simulink model "nid_cvst_what_nid_see"  (Simulink 10.0)
settings: Solver=FixedStepDiscrete  StartTime=0.0  StopTime=inf  RelTol=1e-3  EnableMultiTasking=on
libraries: nid_lib x5, viptextngfix x4, vipsnks x1
settings Model: Creator=tchikama  LastModifiedBy=bhisma
settings DataIOCC: LimitDataPoints=on  SignalLoggingSaveFormat=ModelDataLogs  SaveOutput=off
settings OptimizationCC: ExpressionDepthLimit=2147483647  SimCompilerOptimization=on
settings DebuggingCC: SolverPrmCheckMsg=warning  FcnCallInpInsideContextMsg=warning  StateNameClashWarn=warning
settings HardwareCC: ProdIntDivRoundTo=Zero  ProdEndianess=LittleEndian  ProdHWDeviceType=Generic->32-bit x86 compatible
settings RTWCC: RTWCompilerOptimization=on
settings CodeAppCC: MaxIdLength=95
settings GRTTargetCC: GeneratePreprocessorConditionals=Disable all
settings ConfigComp: CovExternalEMLEnable=off

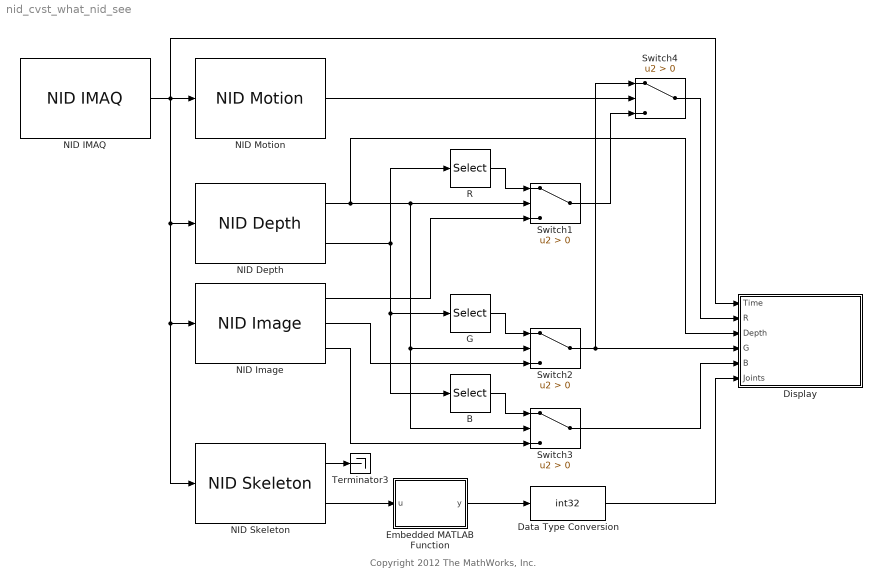
== system nid_cvst_what_nid_see ==
  note: Copyright 2012 The MathWorks, Inc.
  B : Selector  NumberOfDimensions=3  InputPortWidth=3  IndexOptions=Select all,Select all,Index vector (dialog)  Indices=1,2,3  OutputSizes=1,1,1
  Data Type Conversion : DataTypeConversion  OutDataTypeStr=int32
  Display : Subsystem  mask{text_color=[0 0 0]}
      mask prompts: text_color "Text Color (RGB)"
  Embedded MATLAB Function : MATLAB Function  TreatAsAtomicUnit=on
  G : Selector  NumberOfDimensions=3  InputPortWidth=3  IndexOptions=Select all,Select all,Index vector (dialog)  Indices=1,2,2  OutputSizes=1,1,1
  NID Depth : nid_lib/NID Depth  depthOutput=Depth  conv_XYZ_RW=off  viewer=on
  NID IMAQ : nid_lib/NID IMAQ  imaq_depth=on  imaq_motion=on  imaq_image=on  view_point=on  imaq_skeleton=on  imaq_ir=off  mirror_image=off  imaq_sample_time=1/30  res_fps=VGA (640x480): 30 FPS  needPsiPose=off  angle=0  angle_read=off  near_mode=off
  NID Image : nid_lib/NID Image  imageOutput=R/G/B
  NID Motion : nid_lib/NID Motion  viewer=off
  NID Skeleton : nid_lib/NID Skeleton  num_of_skeleton_tracking=1  conv_XYZ_RW=off  viewer=off
  R : Selector  NumberOfDimensions=3  InputPortWidth=3  IndexOptions=Select all,Select all,Index vector (dialog)  Indices=1,2,1  OutputSizes=1,1,1
  Switch{1..4} (4 alike) : Switch  Criteria=u2 > Threshold
  Terminator3 : Terminator
  wires:
  NID IMAQ/1 -> NID Motion/1, NID Depth/1, NID Skeleton/1, NID Image/1, Display/1(Time)
  R/1 -> Switch1/1
  NID Image/1 -> Switch1/3
  G/1 -> Switch2/1
  B/1 -> Switch3/1
  NID Image/2 -> Switch2/3
  NID Image/3 -> Switch3/3
  NID Depth/2 -> R/1, G/1, B/1
  NID Depth/1 -> Switch1/2, Switch2/2, Switch3/2, Display/3(Depth)
  Switch2/1 -> Switch4/1, Display/4(G)
  NID Motion/1 -> Switch4/2
  Switch1/1 -> Switch4/3
  Switch4/1 -> Display/2(R)
  Switch3/1 -> Display/5(B)
  NID Skeleton/1 -> Terminator3/1
  NID Skeleton/2 -> Embedded MATLAB Function/1(u)
  Embedded MATLAB Function/1(y) -> Data Type Conversion/1
  Data Type Conversion/1 -> Display/6(Joints)

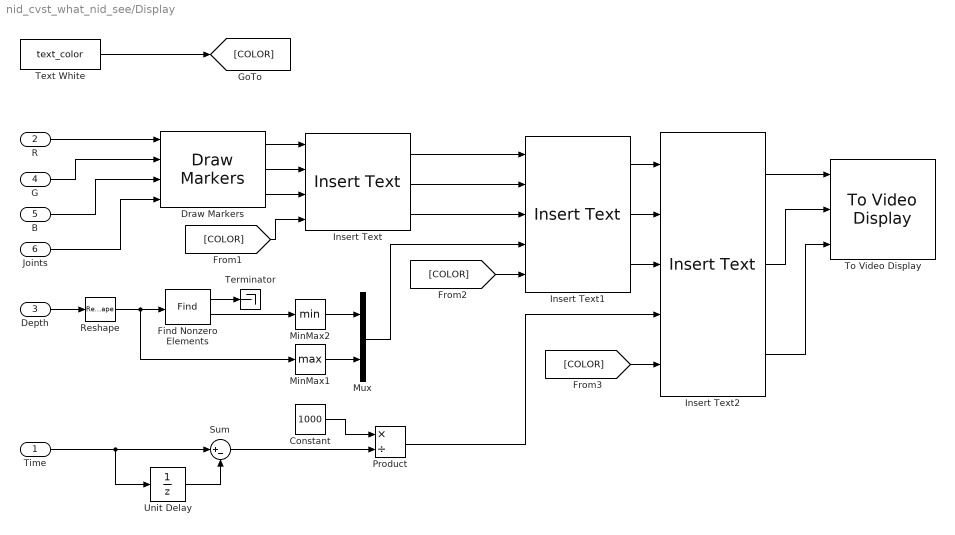
== system nid_cvst_what_nid_see/Display ==
  Time : Inport
  R : Inport  Port=2
  Depth : Inport  Port=3
  G : Inport  Port=4
  B : Inport  Port=5
  Joints : Inport  Port=6
  Constant : Constant  Value=1000
  Draw Markers : viptextngfix/Draw Markers  shape=Circle  size=5  fill=on  fillClrSource=Specify via dialog  display=User-specified value  intensity=200  color=[255 0 0]  opacity=0.5  viewport=Entire image  antialiasing=on  inType=Obsolete  imagePorts=Separate color signals  prodOutputMode=Binary point scaling  prodOutputWordLength=32  prodOutputFracLength=14  memoryMode=Specify word length  memoryWordLength=16  memoryFracLength=14  roundingMode=Floor  overflowMode=off
      settings: SourceProductName=Computer Vision Toolbox  SourceProductBaseCode=VP
  Find Nonzero Elements : Find  NumberOfInputDimensions=3  IndexMode=Zero-based  ShowOutputForNonzeroInputValues=on
  Insert Text : viptextngfix/Insert Text  inputType=Obsolete  theText='RGB camera + Depth (Green) + Motion (Yellow) + Skeleton Joints(Red)'  fontFace=Arial  dummyVar1=0  blockFontSize=16  antiAliased=on  getTextLocFrom=Specify via dialog  textLoc=[0 0]  getTextColorFrom=Input port  textColor=[0 0 0]  getTextIntensityFrom=Specify via dialog  textIntensity=0  getTextOpacityFrom=Specify via dialog  textOpacity=1.0  dummyVar2=0  dummyVar3=0  dummyVar4=0  imagePorts=Separate color signals  isInputTransposed=off
      settings: SourceProductName=Computer Vision Toolbox  SourceProductBaseCode=VP
  Insert Text1 : viptextngfix/Insert Text  inputType=Obsolete  theText='Near: %4.2f[m] Far: %4.2f[m]'  fontFace=Arial  dummyVar1=0  blockFontSize=16  antiAliased=on  getTextLocFrom=Specify via dialog  textLoc=[20 0]  getTextColorFrom=Input port  textColor=[0 0 0]  getTextIntensityFrom=Specify via dialog  textIntensity=0  getTextOpacityFrom=Specify via dialog  textOpacity=1.0  dummyVar2=0  dummyVar3=0  dummyVar4=0  imagePorts=Separate color signals  isInputTransposed=off
      settings: SourceProductName=Computer Vision Toolbox  SourceProductBaseCode=VP
  Insert Text2 : viptextngfix/Insert Text  inputType=Obsolete  theText='%2.0f [FPS]'  fontFace=Arial  dummyVar1=0  blockFontSize=16  antiAliased=on  getTextLocFrom=Specify via dialog  textLoc=[40 0]  getTextColorFrom=Input port  textColor=[0 0 0]  getTextIntensityFrom=Specify via dialog  textIntensity=0  getTextOpacityFrom=Specify via dialog  textOpacity=1.0  dummyVar2=0  dummyVar3=0  dummyVar4=0  imagePorts=Separate color signals  isInputTransposed=off
      settings: SourceProductName=Computer Vision Toolbox  SourceProductBaseCode=VP
  MinMax1 : MinMax  Function=max
  MinMax2 : MinMax
  Mux : Mux  Inputs=2
  Product : Product  Inputs=*/  RndMeth=Zero
  Reshape : Reshape
  Sum : Sum  Inputs=|+-
  Terminator : Terminator
  Text White : Constant  Value=text_color  OutDataTypeStr=uint8
  To Video Display : vipsnks/To Video Display  inputType=Obsolete  imagePorts=Separate color signals  OutputDevice=On-screen video monitor  fullScreen=off  videoWindowX=105  videoWindowY=22  saveWindowSize=off  videoWindowWidth=640  videoWindowHeight=480  dataOrg=Column-major  openAtMdlStart=on  isWindowOpen=on
      settings: SourceProductName=Computer Vision Toolbox  SourceProductBaseCode=VP
  Unit Delay : UnitDelay  SampleTime=-1
  wires:
  Draw Markers/1 -> Insert Text/1
  Draw Markers/2 -> Insert Text/2
  Draw Markers/3 -> Insert Text/3
  R/1 -> Draw Markers/1
  G/1 -> Draw Markers/2
  B/1 -> Draw Markers/3
  Joints/1 -> Draw Markers/4
  Depth/1 -> Reshape/1
  Reshape/1 -> Find Nonzero Elements/1, MinMax1/1
  Find Nonzero Elements/2 -> MinMax2/1
  Find Nonzero Elements/1 -> Terminator/1
  MinMax2/1 -> Mux/1
  MinMax1/1 -> Mux/2
  Insert Text/1 -> Insert Text1/1
  Insert Text/2 -> Insert Text1/2
  Mux/1 -> Insert Text1/4
  Time/1 -> Sum/1, Unit Delay/1
  Unit Delay/1 -> Sum/2
  Constant/1 -> Product/1
  Sum/1 -> Product/2
  Insert Text1/1 -> Insert Text2/1
  Insert Text1/2 -> Insert Text2/2
  Insert Text1/3 -> Insert Text2/3
  Product/1 -> Insert Text2/4
  Insert Text2/1 -> To Video Display/1
  Insert Text/3 -> Insert Text1/3
  Insert Text2/2 -> To Video Display/2
  Insert Text2/3 -> To Video Display/3
  Text White/1 -> [COLOR]
  [COLOR] -> Insert Text/4
  [COLOR] -> Insert Text1/5
  [COLOR] -> Insert Text2/5

== matlab function Embedded MATLAB Function ==
  data: u input double; y output double
function y = fcn(u)
%#eml

jointSize = size(u); 
tmp = zeros(2, jointSize(2));

for i = 1:jointSize(2)
    tmp(1,i) = u(1,i,2);
    tmp(2,i) = u(1,i,1);
end

y = tmp;
